simulink model "BGOnly2"  (R2017b)
settings: Solver=VariableStepAuto  StartTime=0.0  StopTime=60  RelTol=1e-3  EnableMultiTasking=on
values from neighbouring files (symbols this model uses):
  beta_str_ch = 0.5*ones(1,5)    [BGOnly2SwitchTest.m]    (also in BGOnlyVar.mat = [0.5 0.5 0.5 0.5 0.5]; PlotBGOnly2.m)
  nu_gpe = 1    [BGOnlyVar.mat]
  nu_gpi = 1    [BGOnlyVar.mat]
  nu_stn = 1    [BGOnlyVar.mat]
  nu_str = 1    [BGOnlyVar.mat]
  teta = 0.02    [BGOnlyVar.mat]
  w_e = 0.9    [BGOnlyVar.mat]
  w_g = 1    [BGOnlyVar.mat]
  w_inh = 0    [BGOnlyVar.mat]
  w_minus = 1    [BGOnlyVar.mat]
  w_plus = 0.9    [BGOnlyVar.mat]
  w_s = 1    [BGOnlyVar.mat]
  w_t = 0.9    [BGOnlyVar.mat]
undefined symbols (not defined in the file or in its folder): sigbuilder_block
libraries: fuzblock x25, simulink x8
settings Model: Creator=User  LastModifiedBy=acaso
settings DataIOCC: LimitDataPoints=on
settings OptimizationCC: LifeSpan=inf
settings DebuggingCC: AllowSymbolicDim=off  SFUnexpectedBacktrackingDiag=warning  SFNoUnconditionalDefaultTransitionDiag=warning  SFExecutionAtInitializationDiag=none
settings ModelReferenceCC: PropagateSignalLabelsOutOfModel=off
settings CodeAppCC: StateflowObjectComments=on
settings GRTTargetCC: TargetLangStandard=C89/C90 (ANSI)
settings ConfigComp: CovMetricSettings=dw  CovHtmlReporting=on  CovSaveCumulativeToWorkspaceVar=on  CovSaveSingleToWorkspaceVar=on  CovExternalEMLEnable=off

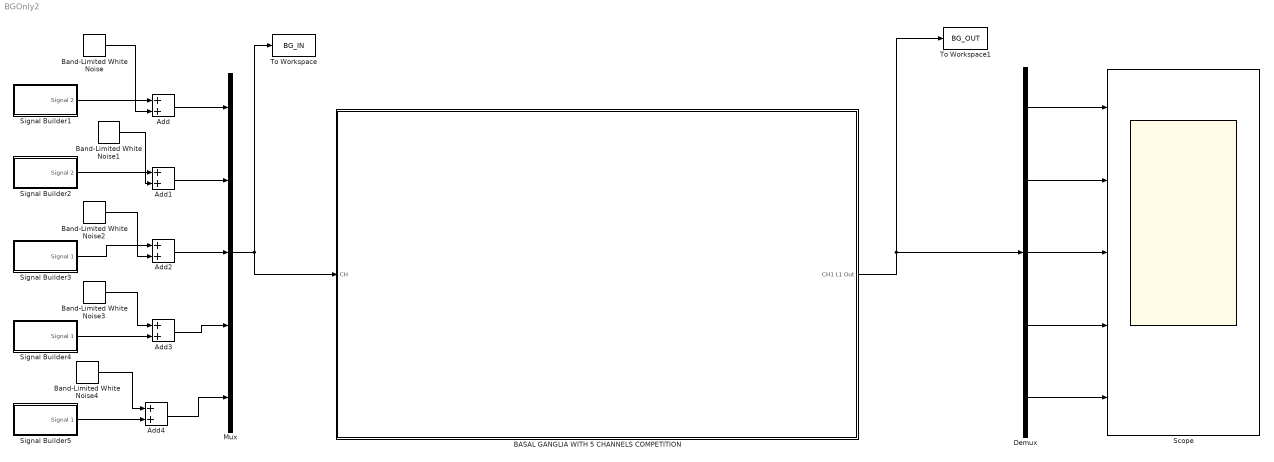
== system BGOnly2 ==
  Add{,1..4} (5 alike) : Sum
  BASAL GANGLIA WITH 5 CHANNELS COMPETITION : Subsystem
  Band-Limited White Noise{,1..4} (5 alike) : simulink/Sources/Band-Limited White Noise  Cov=CHNoise  Ts=0.1  seed=[23341]
  Demux : Demux  Outputs=5
  Mux : Mux  Inputs=5
  Scope : Scope  NumInputPorts=5
  Signal Builder1 : Subsystem  Tag=STV Subsys  LoadFcn=sigbuilder_block('load');  StartFcn=sigbuilder_block('start');  StopFcn=sigbuilder_block('stop');  ClipboardFcn=sigbuilder_block('clipboard');  mask(Sigbuilder block){tuvar=[0:10]}
      mask help: Simulink:masks:SigbuilderBlock_MD
      mask init:
      | if ~strcmp(get_param(bdroot(gcbh),'SimulationStatus'),'stopped') tuvar = sigbuilder_block('maskInit'); end
      settings: CopyFcn=sigbuilder_block('copy');  DeleteFcn=sigbuilder_block('delete');  ModelCloseFcn=sigbuilder_block('modelClose');  PreSaveFcn=sigbuilder_block('preSave');  PauseFcn=sigbuilder_block('pause');  ContinueFcn=sigbuilder_block('continue');  NameChangeFcn=sigbuilder_block('namechange');  OpenFcn=sigbuilder_block('open',[5.4 60.6 1141.2 492 ]);  CloseFcn=sigbuilder_block('close');
      mask Display: plot(0, 0, 100, 100,[2, 2, 32, 32, 2], [68, 8, 8, 68, 68],[32, 2], [38, 38], [32, 19, 2],[53, 60, 44], [32, 17, 17, 2],[16, 16, 31, 31]);txt = getActiveGroup(gcbh);text(2, 100, txt,'verticalAlignment', 'top');
  Signal Builder2 : Subsystem  Tag=STV Subsys  LoadFcn=sigbuilder_block('load');  StartFcn=sigbuilder_block('start');  StopFcn=sigbuilder_block('stop');  ClipboardFcn=sigbuilder_block('clipboard');  mask(Sigbuilder block){tuvar=[0:10]}
      mask help: Simulink:masks:SigbuilderBlock_MD
      mask init:
      | if ~strcmp(get_param(bdroot(gcbh),'SimulationStatus'),'stopped') tuvar = sigbuilder_block('maskInit'); end
      settings: CopyFcn=sigbuilder_block('copy');  DeleteFcn=sigbuilder_block('delete');  ModelCloseFcn=sigbuilder_block('modelClose');  PreSaveFcn=sigbuilder_block('preSave');  PauseFcn=sigbuilder_block('pause');  ContinueFcn=sigbuilder_block('continue');  NameChangeFcn=sigbuilder_block('namechange');  OpenFcn=sigbuilder_block('open',[223.8 139.8 727.2 446.4 ]);  CloseFcn=sigbuilder_block('close');
      mask Display: plot(0, 0, 100, 100,[2, 2, 32, 32, 2], [68, 8, 8, 68, 68],[32, 2], [38, 38], [32, 19, 2],[53, 60, 44], [32, 17, 17, 2],[16, 16, 31, 31]);txt = getActiveGroup(gcbh);text(2, 100, txt,'verticalAlignment', 'top');
  Signal Builder3 : Subsystem  Tag=STV Subsys  LoadFcn=sigbuilder_block('load');  StartFcn=sigbuilder_block('start');  StopFcn=sigbuilder_block('stop');  ClipboardFcn=sigbuilder_block('clipboard');  mask(Sigbuilder block){tuvar=[0:10]}
      mask help: Simulink:masks:SigbuilderBlock_MD
      mask init:
      | if ~strcmp(get_param(bdroot(gcbh),'SimulationStatus'),'stopped') tuvar = sigbuilder_block('maskInit'); end
      settings: CopyFcn=sigbuilder_block('copy');  DeleteFcn=sigbuilder_block('delete');  ModelCloseFcn=sigbuilder_block('modelClose');  PreSaveFcn=sigbuilder_block('preSave');  PauseFcn=sigbuilder_block('pause');  ContinueFcn=sigbuilder_block('continue');  NameChangeFcn=sigbuilder_block('namechange');  OpenFcn=sigbuilder_block('open',[216.6 86.4 727.8 484.8 ]);  CloseFcn=sigbuilder_block('close');
      mask Display: plot(0, 0, 100, 100,[2, 2, 32, 32, 2], [68, 8, 8, 68, 68],[32, 2], [38, 38], [32, 19, 2],[53, 60, 44], [32, 17, 17, 2],[16, 16, 31, 31]);txt = getActiveGroup(gcbh);text(2, 100, txt,'verticalAlignment', 'top');
  Signal Builder4 : Subsystem  Tag=STV Subsys  LoadFcn=sigbuilder_block('load');  StartFcn=sigbuilder_block('start');  StopFcn=sigbuilder_block('stop');  ClipboardFcn=sigbuilder_block('clipboard');  mask(Sigbuilder block){tuvar=[0:10]}
      mask help: Simulink:masks:SigbuilderBlock_MD
      mask init:
      | if ~strcmp(get_param(bdroot(gcbh),'SimulationStatus'),'stopped') tuvar = sigbuilder_block('maskInit'); end
      settings: CopyFcn=sigbuilder_block('copy');  DeleteFcn=sigbuilder_block('delete');  ModelCloseFcn=sigbuilder_block('modelClose');  PreSaveFcn=sigbuilder_block('preSave');  PauseFcn=sigbuilder_block('pause');  ContinueFcn=sigbuilder_block('continue');  NameChangeFcn=sigbuilder_block('namechange');  OpenFcn=sigbuilder_block('open',[216.75 86.25 727.5 485.25 ]);  CloseFcn=sigbuilder_block('close');
      mask Display: plot(0, 0, 100, 100,[2, 2, 32, 32, 2], [68, 8, 8, 68, 68],[32, 2], [38, 38], [32, 19, 2],[53, 60, 44], [32, 17, 17, 2],[16, 16, 31, 31]);txt = getActiveGroup(gcbh);text(2, 100, txt,'verticalAlignment', 'top');
  Signal Builder5 : Subsystem  Tag=STV Subsys  LoadFcn=sigbuilder_block('load');  StartFcn=sigbuilder_block('start');  StopFcn=sigbuilder_block('stop');  ClipboardFcn=sigbuilder_block('clipboard');  mask(Sigbuilder block){tuvar=[0:10]}
      mask help: Simulink:masks:SigbuilderBlock_MD
      mask init:
      | if ~strcmp(get_param(bdroot(gcbh),'SimulationStatus'),'stopped') tuvar = sigbuilder_block('maskInit'); end
      settings: CopyFcn=sigbuilder_block('copy');  DeleteFcn=sigbuilder_block('delete');  ModelCloseFcn=sigbuilder_block('modelClose');  PreSaveFcn=sigbuilder_block('preSave');  PauseFcn=sigbuilder_block('pause');  ContinueFcn=sigbuilder_block('continue');  NameChangeFcn=sigbuilder_block('namechange');  OpenFcn=sigbuilder_block('open',[216.75 86.25 727.5 485.25 ]);  CloseFcn=sigbuilder_block('close');
      mask Display: plot(0, 0, 100, 100,[2, 2, 32, 32, 2], [68, 8, 8, 68, 68],[32, 2], [38, 38], [32, 19, 2],[53, 60, 44], [32, 17, 17, 2],[16, 16, 31, 31]);txt = getActiveGroup(gcbh);text(2, 100, txt,'verticalAlignment', 'top');
  To Workspace : ToWorkspace  VariableName=BG_IN  SaveFormat=Timeseries  SampleTime=0.1
  To Workspace1 : ToWorkspace  VariableName=BG_OUT  SaveFormat=Timeseries  SampleTime=0.1
  wires:
  Mux/1 -> To Workspace/1, BASAL GANGLIA WITH 5 CHANNELS COMPETITION/1("CH ")
  BASAL GANGLIA WITH 5 CHANNELS COMPETITION/1(CH1 L1 Out) -> To Workspace1/1, Demux/1
  Demux/5 -> Scope/5
  Demux/4 -> Scope/4
  Demux/3 -> Scope/3
  Demux/2 -> Scope/2
  Demux/1 -> Scope/1
  Signal Builder1/1(Signal 2) -> Add/1
  Add/1 -> Mux/1
  Band-Limited White Noise/1 -> Add/2
  Add1/1 -> Mux/2
  Signal Builder2/1(Signal 2) -> Add1/1
  Band-Limited White Noise1/1 -> Add1/2
  Add2/1 -> Mux/3
  Signal Builder3/1(Signal 1) -> Add2/1
  Band-Limited White Noise2/1 -> Add2/2
  Add3/1 -> Mux/4
  Signal Builder4/1(Signal 1) -> Add3/2
  Band-Limited White Noise3/1 -> Add3/1
  Add4/1 -> Mux/5
  Signal Builder5/1(Signal 1) -> Add4/2
  Band-Limited White Noise4/1 -> Add4/1

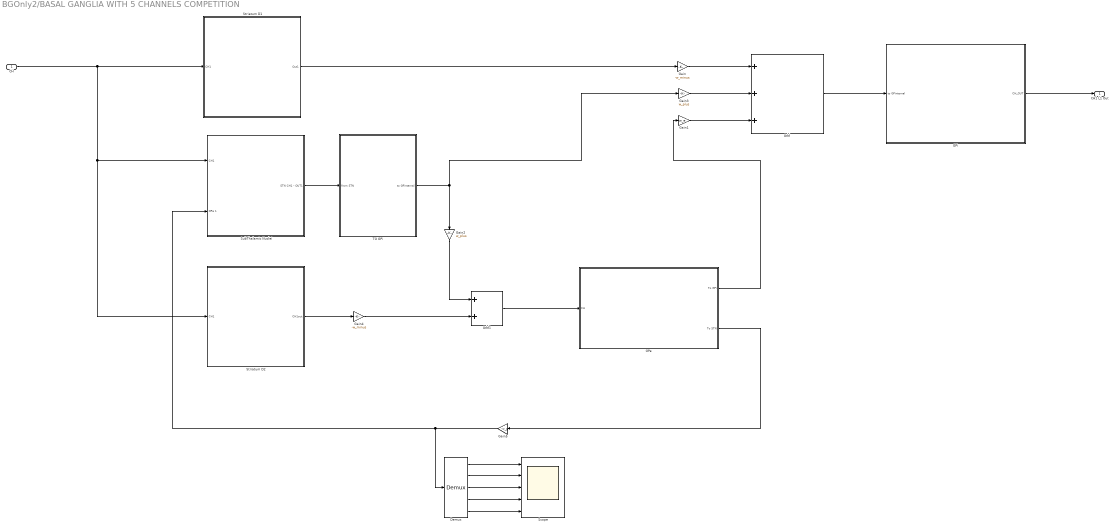
== system BGOnly2/BASAL GANGLIA WITH 5 CHANNELS COMPETITION ==
  "CH " : Inport
  Add : Sum  Inputs=3
  Add1 : Sum  Inputs=2
  Demux : Demux  Outputs=5
  GPe : Subsystem  TreatAsAtomicUnit=on
  GPi : Subsystem
  Gain : Gain  Gain=-w_minus
  Gain1 : Gain  Gain=w_e
  Gain2 : Gain  Gain=w_plus
  Gain3 : Gain  Gain=w_plus
  Gain4 : Gain  Gain=-w_minus
  Gain5 : Gain  Gain=-w_g
  Scope : Scope  NumInputPorts=5
  "Striatum D1 " : Subsystem
  Striatum D2 : Subsystem
  SubThalamic Nuclei : Subsystem
  TO GPi : Subsystem
  CH1 L1 Out : Outport
  wires:
  TO GPi/1(to GPinternal) -> Gain3/1, Gain2/1
  GPi/1("CH_OUT ") -> CH1 L1 Out/1
  "CH "/1 -> Striatum D2/1(CH1), SubThalamic Nuclei/1(CH1), "Striatum D1 "/1(CH1)
  "Striatum D1 "/1(Out1) -> Gain/1
  SubThalamic Nuclei/1(STN CH1 - OUT1) -> TO GPi/1("from STN ")
  GPe/1(To GPi) -> Gain1/1
  Gain/1 -> Add/1
  Gain3/1 -> Add/2
  Gain1/1 -> Add/3
  Striatum D2/1(CH1out) -> Gain4/1
  Gain2/1 -> Add1/1
  Gain4/1 -> Add1/2
  Add1/1 -> GPe/1(CH)
  GPe/2(To STN) -> Gain5/1
  Gain5/1 -> Demux/1, SubThalamic Nuclei/2(GPe 1)
  Add/1 -> GPi/1("to GPinternal ")
  Demux/1 -> Scope/1
  Demux/2 -> Scope/2
  Demux/3 -> Scope/3
  Demux/4 -> Scope/4
  Demux/5 -> Scope/5

== system BGOnly2/Signal Builder1 ==
  Demux : Demux  Tag=STV Demux  Outputs=1
  FromWs : FromWorkspace  Tag=STV FromWs  VariableName=tuvar  SampleTime=0
      SigBuilderData=|
      | common.afterFinalStr = 'Extrapolate'
      | common.sampleTime = 0
      | dataSet.timeRange = [0 60]
      | dataSet.name = 'Group 1'
      | sbobj.Groups.Name = 'Group 1'
      | sbobj.Groups.Signals.Name = 'Signal 2'
      | sbobj.Groups.Signals.XData = [0 20.1 20.1 29.5 30.4 40.1 40.1 59.7 60]
      | sbobj.Groups.Signals.YData = [0 0 1 1 0.8 0.795 0.005 0.0001 0.0001]
      | sbobj.Groups.TimeRange = [0 60]
  Signal 2 : Outport  Tag=STV Outport
  wires:
  FromWs/1 -> Demux/1
  Demux/1 -> Signal 2/1

== system BGOnly2/Signal Builder2 ==
  Demux : Demux  Tag=STV Demux  Outputs=1
  FromWs : FromWorkspace  Tag=STV FromWs  VariableName=tuvar  SampleTime=0
      SigBuilderData=|
      | common.afterFinalStr = 'Extrapolate'
      | common.sampleTime = 0
      | dataSet.timeRange = [0 60]
      | dataSet.name = 'Group 1'
      | sbobj.Groups.Name = 'Group 1'
      | sbobj.Groups.Signals.Name = 'Signal 2'
      | sbobj.Groups.Signals.XData = [0 30.1 30.1 39.7 40.4 49.9 49.9 60]
      | sbobj.Groups.Signals.YData = [0 0 0.8 0.795 1 1 0 0]
      | sbobj.Groups.TimeRange = [0 60]
  Signal 2 : Outport  Tag=STV Outport
  wires:
  FromWs/1 -> Demux/1
  Demux/1 -> Signal 2/1

== system BGOnly2/Signal Builder3 ==
  Demux : Demux  Tag=STV Demux  Outputs=1
  FromWs : FromWorkspace  Tag=STV FromWs  VariableName=tuvar  SampleTime=0
      SigBuilderData=|
      | common.afterFinalStr = 'Extrapolate'
      | common.sampleTime = 0
      | dataSet.timeRange = [0 60]
      | dataSet.name = 'Group 1'
      | sbobj.Groups.Name = 'Group 1'
      | sbobj.Groups.Signals.Name = 'Signal 1'
      | sbobj.Groups.Signals.XData = [0 60]
      | sbobj.Groups.Signals.YData = [0 0]
      | sbobj.Groups.TimeRange = [0 60]
  Signal 1 : Outport  Tag=STV Outport
  wires:
  FromWs/1 -> Demux/1
  Demux/1 -> Signal 1/1

== system BGOnly2/Signal Builder4 ==
  Demux : Demux  Tag=STV Demux  Outputs=1
  FromWs : FromWorkspace  Tag=STV FromWs  VariableName=tuvar  SampleTime=0
      SigBuilderData=|
      | common.afterFinalStr = 'Extrapolate'
      | common.sampleTime = 0
      | dataSet.timeRange = [0 60]
      | dataSet.name = 'Group 1'
      | sbobj.Groups.Name = 'Group 1'
      | sbobj.Groups.Signals.Name = 'Signal 1'
      | sbobj.Groups.Signals.XData = [0 60]
      | sbobj.Groups.Signals.YData = [0 0]
      | sbobj.Groups.TimeRange = [0 60]
  Signal 1 : Outport  Tag=STV Outport
  wires:
  FromWs/1 -> Demux/1
  Demux/1 -> Signal 1/1

== system BGOnly2/Signal Builder5 ==
  Demux : Demux  Tag=STV Demux  Outputs=1
  FromWs : FromWorkspace  Tag=STV FromWs  VariableName=tuvar  SampleTime=0
      SigBuilderData=|
      | common.afterFinalStr = 'Extrapolate'
      | common.sampleTime = 0
      | dataSet.timeRange = [0 60]
      | dataSet.name = 'Group 1'
      | sbobj.Groups.Name = 'Group 1'
      | sbobj.Groups.Signals.Name = 'Signal 1'
      | sbobj.Groups.Signals.XData = [0 60]
      | sbobj.Groups.Signals.YData = [0 0]
      | sbobj.Groups.TimeRange = [0 60]
  Signal 1 : Outport  Tag=STV Outport
  wires:
  FromWs/1 -> Demux/1
  Demux/1 -> Signal 1/1

== system BGOnly2/BASAL GANGLIA WITH 5 CHANNELS COMPETITION/GPe ==
  CH : Inport
  GPe CH1 : Subsystem
  To GPi : Outport
  To STN : Outport  Port=2
  wires:
  CH/1 -> GPe CH1/1(In)
  GPe CH1/1(To GPi) -> To GPi/1
  GPe CH1/2(To STN) -> To STN/1

== system BGOnly2/BASAL GANGLIA WITH 5 CHANNELS COMPETITION/GPi ==
  "to GPinternal " : Inport
  GPinternal : Subsystem
  "CH_OUT " : Outport
  wires:
  "to GPinternal "/1 -> GPinternal/1("to GPinternal ")
  GPinternal/1(To Thal) -> "CH_OUT "/1

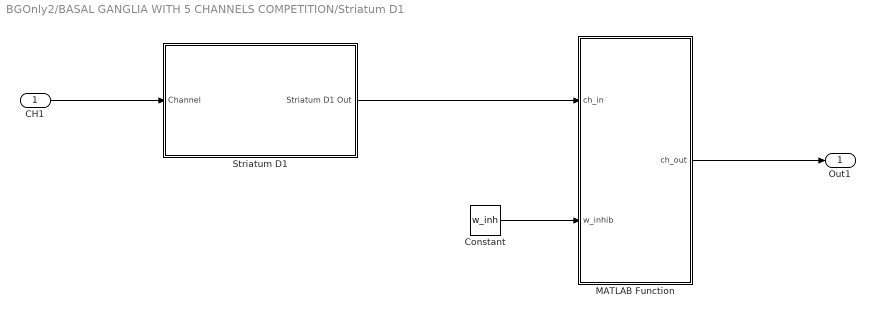
== system BGOnly2/BASAL GANGLIA WITH 5 CHANNELS COMPETITION/Striatum D1  ==
  CH1 : Inport
  Constant : Constant  Value=w_inh
  MATLAB Function : MATLAB Function  TreatAsAtomicUnit=on
  "Striatum D1 " : Subsystem
  Out1 : Outport
  wires:
  CH1/1 -> "Striatum D1 "/1(Channel)
  "Striatum D1 "/1(Striatum D1 Out) -> MATLAB Function/1(ch_in)
  Constant/1 -> MATLAB Function/2(w_inhib)
  MATLAB Function/1(ch_out) -> Out1/1

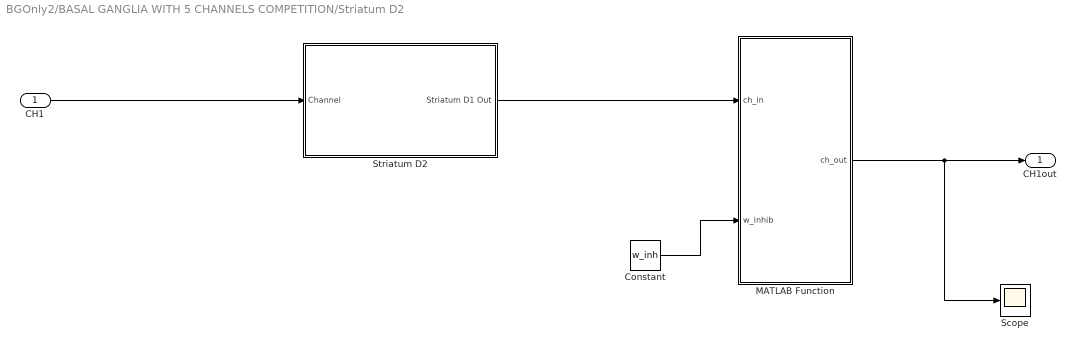
== system BGOnly2/BASAL GANGLIA WITH 5 CHANNELS COMPETITION/Striatum D2 ==
  CH1 : Inport
  Constant : Constant  Value=w_inh
  MATLAB Function : MATLAB Function  TreatAsAtomicUnit=on
  Scope : Scope
  "Striatum D2 " : Subsystem
  CH1out : Outport
  wires:
  MATLAB Function/1(ch_out) -> Scope/1, CH1out/1
  CH1/1 -> "Striatum D2 "/1(Channel)
  "Striatum D2 "/1(Striatum D1 Out) -> MATLAB Function/1(ch_in)
  Constant/1 -> MATLAB Function/2(w_inhib)

== system BGOnly2/BASAL GANGLIA WITH 5 CHANNELS COMPETITION/SubThalamic Nuclei ==
  CH1 : Inport
  GPe 1 : Inport  Port=2
  "SubThalamic Nucleus (STN) " : Subsystem
  STN CH1 - OUT1 : Outport
  wires:
  CH1/1 -> "SubThalamic Nucleus (STN) "/1(Channel)
  GPe 1/1 -> "SubThalamic Nucleus (STN) "/2(GPe Inp)
  "SubThalamic Nucleus (STN) "/1(STN Out1) -> STN CH1 - OUT1/1

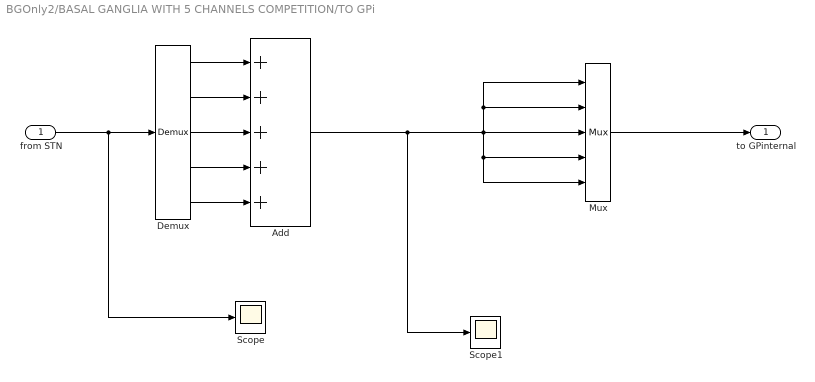
== system BGOnly2/BASAL GANGLIA WITH 5 CHANNELS COMPETITION/TO GPi ==
  "from STN " : Inport
  Add : Sum  Inputs=5
  Demux : Demux  Outputs=5
  Mux : Mux  Inputs=5
  Scope : Scope
  Scope1 : Scope
  to GPinternal : Outport
  wires:
  "from STN "/1 -> Scope/1, Demux/1
  Demux/1 -> Add/1
  Demux/2 -> Add/2
  Demux/3 -> Add/3
  Demux/4 -> Add/4
  Demux/5 -> Add/5
  Add/1 -> Scope1/1, Mux/1, Mux/2, Mux/3, Mux/4, Mux/5
  Mux/1 -> to GPinternal/1

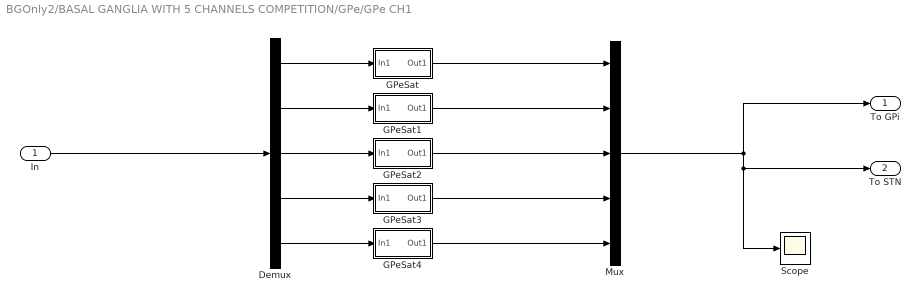
== system BGOnly2/BASAL GANGLIA WITH 5 CHANNELS COMPETITION/GPe/GPe CH1 ==
  In : Inport
  Demux : Demux  Outputs=5
  GPeSat : Subsystem
  GPeSat1 : Subsystem
  GPeSat2 : Subsystem
  GPeSat3 : Subsystem
  GPeSat4 : Subsystem
  Mux : Mux  Inputs=5
  Scope : Scope
  To GPi : Outport
  To STN : Outport  Port=2
  wires:
  Mux/1 -> To STN/1, Scope/1, To GPi/1
  Demux/1 -> GPeSat/1(In1)
  GPeSat/1(Out1) -> Mux/1
  Demux/2 -> GPeSat1/1(In1)
  GPeSat1/1(Out1) -> Mux/2
  Demux/3 -> GPeSat2/1(In1)
  GPeSat2/1(Out1) -> Mux/3
  Demux/4 -> GPeSat3/1(In1)
  GPeSat3/1(Out1) -> Mux/4
  Demux/5 -> GPeSat4/1(In1)
  GPeSat4/1(Out1) -> Mux/5
  In/1 -> Demux/1

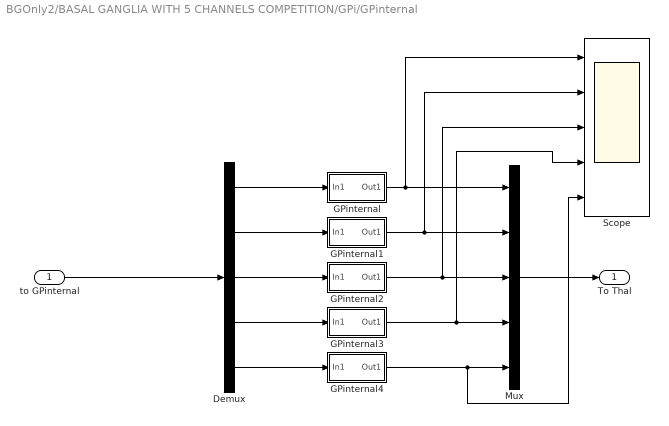
== system BGOnly2/BASAL GANGLIA WITH 5 CHANNELS COMPETITION/GPi/GPinternal ==
  "to GPinternal " : Inport
  Demux : Demux  Outputs=5
  GPinternal : Subsystem
  GPinternal1 : Subsystem
  GPinternal2 : Subsystem
  GPinternal3 : Subsystem
  GPinternal4 : Subsystem
  Mux : Mux  Inputs=5
  Scope : Scope  NumInputPorts=5
  To Thal : Outport
  wires:
  Demux/1 -> GPinternal/1(In1)
  GPinternal/1(Out1) -> Mux/1, Scope/1
  Demux/2 -> GPinternal1/1(In1)
  Demux/3 -> GPinternal2/1(In1)
  GPinternal2/1(Out1) -> Scope/3, Mux/3
  Demux/4 -> GPinternal3/1(In1)
  GPinternal3/1(Out1) -> Scope/4, Mux/4
  Demux/5 -> GPinternal4/1(In1)
  GPinternal4/1(Out1) -> Scope/5, Mux/5
  "to GPinternal "/1 -> Demux/1
  Mux/1 -> To Thal/1
  GPinternal1/1(Out1) -> Scope/2, Mux/2

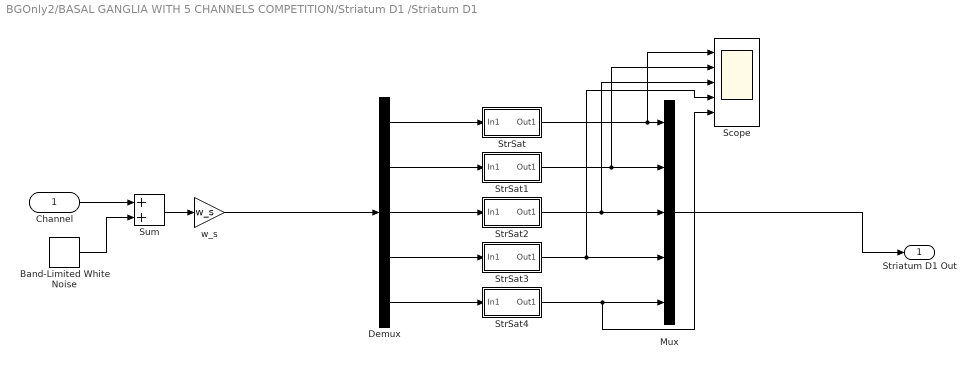
== system BGOnly2/BASAL GANGLIA WITH 5 CHANNELS COMPETITION/Striatum D1 /Striatum D1  ==
  Channel : Inport
  Band-Limited White Noise : simulink/Sources/Band-Limited White Noise  Cov=[0]  Ts=0.1  seed=[23341]
  Demux : Demux  Outputs=5
  Mux : Mux  Inputs=5
  Scope : Scope  NumInputPorts=5
  StrSat : Subsystem
  StrSat1 : Subsystem
  StrSat2 : Subsystem
  StrSat3 : Subsystem
  StrSat4 : Subsystem
  Sum : Sum
  w_s : Gain  Gain=w_s
  Striatum D1 Out : Outport
  wires:
  Channel/1 -> Sum/1
  Sum/1 -> w_s/1
  Mux/1 -> Striatum D1 Out/1
  Band-Limited White Noise/1 -> Sum/2
  Demux/1 -> StrSat/1(In1)
  StrSat/1(Out1) -> Scope/1, Mux/1
  Demux/2 -> StrSat1/1(In1)
  StrSat1/1(Out1) -> Scope/2, Mux/2
  Demux/3 -> StrSat2/1(In1)
  StrSat2/1(Out1) -> Scope/3, Mux/3
  Demux/4 -> StrSat3/1(In1)
  StrSat3/1(Out1) -> Scope/4, Mux/4
  Demux/5 -> StrSat4/1(In1)
  w_s/1 -> Demux/1
  StrSat4/1(Out1) -> Scope/5, Mux/5

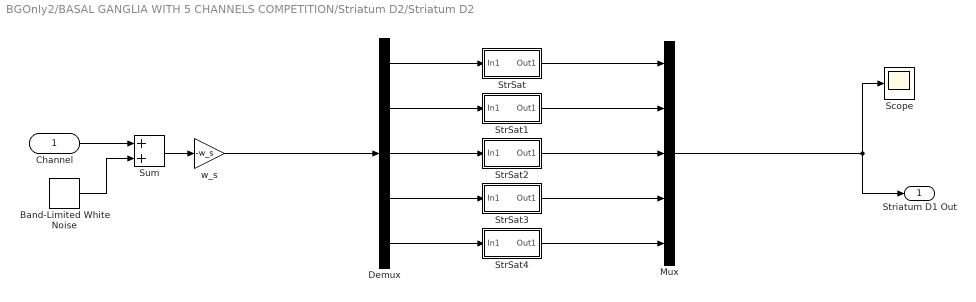
== system BGOnly2/BASAL GANGLIA WITH 5 CHANNELS COMPETITION/Striatum D2/Striatum D2  ==
  Channel : Inport
  Band-Limited White Noise : simulink/Sources/Band-Limited White Noise  Cov=[0]  Ts=0.1  seed=[23341]
  Demux : Demux  Outputs=5
  Mux : Mux  Inputs=5
  Scope : Scope
  StrSat : Subsystem
  StrSat1 : Subsystem
  StrSat2 : Subsystem
  StrSat3 : Subsystem
  StrSat4 : Subsystem
  Sum : Sum
  w_s : Gain  Gain=-w_s
  Striatum D1 Out : Outport
  wires:
  Channel/1 -> Sum/1
  Sum/1 -> w_s/1
  Mux/1 -> Striatum D1 Out/1, Scope/1
  Band-Limited White Noise/1 -> Sum/2
  Demux/1 -> StrSat/1(In1)
  StrSat/1(Out1) -> Mux/1
  Demux/2 -> StrSat1/1(In1)
  StrSat1/1(Out1) -> Mux/2
  Demux/3 -> StrSat2/1(In1)
  StrSat2/1(Out1) -> Mux/3
  Demux/4 -> StrSat3/1(In1)
  StrSat3/1(Out1) -> Mux/4
  Demux/5 -> StrSat4/1(In1)
  StrSat4/1(Out1) -> Mux/5
  w_s/1 -> Demux/1

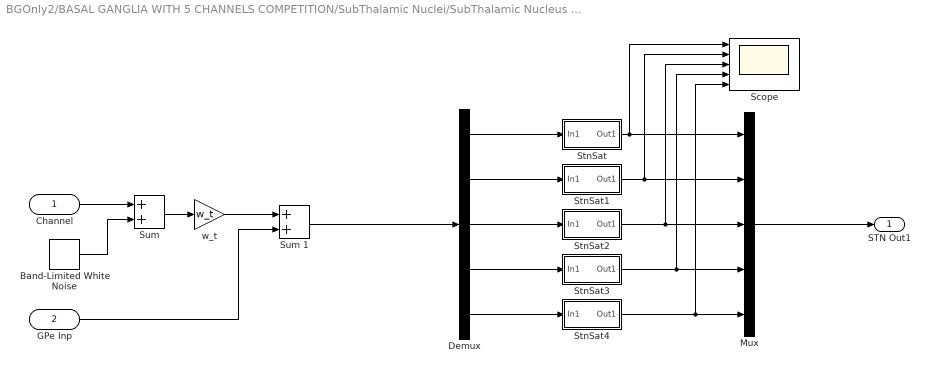
== system BGOnly2/BASAL GANGLIA WITH 5 CHANNELS COMPETITION/SubThalamic Nuclei/SubThalamic Nucleus (STN)  ==
  Channel : Inport
  GPe Inp : Inport  Port=2
  Band-Limited White Noise : simulink/Sources/Band-Limited White Noise  Cov=[0]  Ts=0.1  seed=[23341]
  Demux : Demux  Outputs=5
  Mux : Mux  Inputs=5
  Scope : Scope  NumInputPorts=5
  StnSat : Subsystem
  StnSat1 : Subsystem
  StnSat2 : Subsystem
  StnSat3 : Subsystem
  StnSat4 : Subsystem
  "Sum " : Sum
  Sum 1 : Sum
  w_t : Gain  Gain=w_t
  STN Out1 : Outport
  wires:
  w_t/1 -> Sum 1/1
  Channel/1 -> "Sum "/1
  Band-Limited White Noise/1 -> "Sum "/2
  "Sum "/1 -> w_t/1
  GPe Inp/1 -> Sum 1/2
  Mux/1 -> STN Out1/1
  Demux/1 -> StnSat/1(In1)
  Demux/2 -> StnSat1/1(In1)
  StnSat1/1(Out1) -> Scope/2, Mux/2
  Demux/3 -> StnSat2/1(In1)
  StnSat2/1(Out1) -> Scope/3, Mux/3
  Demux/4 -> StnSat3/1(In1)
  StnSat3/1(Out1) -> Scope/4, Mux/4
  Demux/5 -> StnSat4/1(In1)
  StnSat4/1(Out1) -> Scope/5, Mux/5
  Sum 1/1 -> Demux/1
  StnSat/1(Out1) -> Scope/1, Mux/1

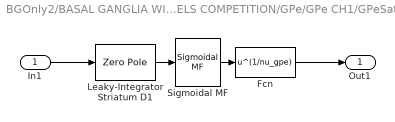
== system BGOnly2/BASAL GANGLIA WITH 5 CHANNELS COMPETITION/GPe/GPe CH1/GPeSat ==
  In1 : Inport
  Fcn : Fcn  Expr=u^(1/nu_gpe)
  "Leaky-Integrator Striatum D1 " : ZeroPole  Zeros=[]  Poles=[-1/teta]  Gain=[1.5/teta]
  Sigmoidal MF : fuzblock/Membership  Functions/Sigmoidal MF  a=alpha_gpe  c=beta_gpe
      settings: SourceProductName=Fuzzy Logic Toolbox  SourceProductBaseCode=FL
  Out1 : Outport
  wires:
  Fcn/1 -> Out1/1
  Sigmoidal MF/1 -> Fcn/1
  "Leaky-Integrator Striatum D1 "/1 -> Sigmoidal MF/1
  In1/1 -> "Leaky-Integrator Striatum D1 "/1

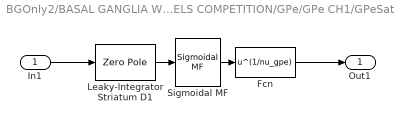
== system BGOnly2/BASAL GANGLIA WITH 5 CHANNELS COMPETITION/GPe/GPe CH1/GPeSat1 ==
  In1 : Inport
  Fcn : Fcn  Expr=u^(1/nu_gpe)
  "Leaky-Integrator Striatum D1 " : ZeroPole  Zeros=[]  Poles=[-1/teta]  Gain=[1.5/teta]
  Sigmoidal MF : fuzblock/Membership  Functions/Sigmoidal MF  a=alpha_gpe  c=beta_gpe
      settings: SourceProductName=Fuzzy Logic Toolbox  SourceProductBaseCode=FL
  Out1 : Outport
  wires:
  Fcn/1 -> Out1/1
  Sigmoidal MF/1 -> Fcn/1
  "Leaky-Integrator Striatum D1 "/1 -> Sigmoidal MF/1
  In1/1 -> "Leaky-Integrator Striatum D1 "/1

== system BGOnly2/BASAL GANGLIA WITH 5 CHANNELS COMPETITION/GPe/GPe CH1/GPeSat2 ==
  In1 : Inport
  Fcn : Fcn  Expr=u^(1/nu_gpe)
  "Leaky-Integrator Striatum D1 " : ZeroPole  Zeros=[]  Poles=[-1/teta]  Gain=[1.5/teta]
  Sigmoidal MF : fuzblock/Membership  Functions/Sigmoidal MF  a=alpha_gpe  c=beta_gpe
      settings: SourceProductName=Fuzzy Logic Toolbox  SourceProductBaseCode=FL
  Out1 : Outport
  wires:
  Fcn/1 -> Out1/1
  Sigmoidal MF/1 -> Fcn/1
  "Leaky-Integrator Striatum D1 "/1 -> Sigmoidal MF/1
  In1/1 -> "Leaky-Integrator Striatum D1 "/1

== system BGOnly2/BASAL GANGLIA WITH 5 CHANNELS COMPETITION/GPe/GPe CH1/GPeSat3 ==
  In1 : Inport
  Fcn : Fcn  Expr=u^(1/nu_gpe)
  "Leaky-Integrator Striatum D1 " : ZeroPole  Zeros=[]  Poles=[-1/teta]  Gain=[1.5/teta]
  Sigmoidal MF : fuzblock/Membership  Functions/Sigmoidal MF  a=alpha_gpe  c=beta_gpe
      settings: SourceProductName=Fuzzy Logic Toolbox  SourceProductBaseCode=FL
  Out1 : Outport
  wires:
  Fcn/1 -> Out1/1
  Sigmoidal MF/1 -> Fcn/1
  "Leaky-Integrator Striatum D1 "/1 -> Sigmoidal MF/1
  In1/1 -> "Leaky-Integrator Striatum D1 "/1

== system BGOnly2/BASAL GANGLIA WITH 5 CHANNELS COMPETITION/GPe/GPe CH1/GPeSat4 ==
  In1 : Inport
  Fcn : Fcn  Expr=u^(1/nu_gpe)
  "Leaky-Integrator Striatum D1 " : ZeroPole  Zeros=[]  Poles=[-1/teta]  Gain=[1.5/teta]
  Sigmoidal MF : fuzblock/Membership  Functions/Sigmoidal MF  a=alpha_gpe  c=beta_gpe
      settings: SourceProductName=Fuzzy Logic Toolbox  SourceProductBaseCode=FL
  Out1 : Outport
  wires:
  Fcn/1 -> Out1/1
  Sigmoidal MF/1 -> Fcn/1
  "Leaky-Integrator Striatum D1 "/1 -> Sigmoidal MF/1
  In1/1 -> "Leaky-Integrator Striatum D1 "/1

== system BGOnly2/BASAL GANGLIA WITH 5 CHANNELS COMPETITION/GPi/GPinternal/GPinternal ==
  In1 : Inport
  Fcn : Fcn  Expr=u^(1/nu_gpi)
  "Leaky-Integrator Striatum D1 " : ZeroPole  Zeros=[]  Poles=[-1/teta]  Gain=[1.5/teta]
  Sigmoidal MF : fuzblock/Membership  Functions/Sigmoidal MF  a=alpha_gpi  c=beta_gpi
      settings: SourceProductName=Fuzzy Logic Toolbox  SourceProductBaseCode=FL
  Out1 : Outport
  wires:
  Fcn/1 -> Out1/1
  Sigmoidal MF/1 -> Fcn/1
  "Leaky-Integrator Striatum D1 "/1 -> Sigmoidal MF/1
  In1/1 -> "Leaky-Integrator Striatum D1 "/1

== system BGOnly2/BASAL GANGLIA WITH 5 CHANNELS COMPETITION/GPi/GPinternal/GPinternal1 ==
  In1 : Inport
  Fcn : Fcn  Expr=u^(1/nu_gpi)
  "Leaky-Integrator Striatum D1 " : ZeroPole  Zeros=[]  Poles=[-1/teta]  Gain=[1.5/teta]
  Sigmoidal MF : fuzblock/Membership  Functions/Sigmoidal MF  a=alpha_gpi  c=beta_gpi
      settings: SourceProductName=Fuzzy Logic Toolbox  SourceProductBaseCode=FL
  Out1 : Outport
  wires:
  Fcn/1 -> Out1/1
  Sigmoidal MF/1 -> Fcn/1
  "Leaky-Integrator Striatum D1 "/1 -> Sigmoidal MF/1
  In1/1 -> "Leaky-Integrator Striatum D1 "/1

== system BGOnly2/BASAL GANGLIA WITH 5 CHANNELS COMPETITION/GPi/GPinternal/GPinternal2 ==
  In1 : Inport
  Fcn : Fcn  Expr=u^(1/nu_gpi)
  "Leaky-Integrator Striatum D1 " : ZeroPole  Zeros=[]  Poles=[-1/teta]  Gain=[1.5/teta]
  Sigmoidal MF : fuzblock/Membership  Functions/Sigmoidal MF  a=alpha_gpi  c=beta_gpi
      settings: SourceProductName=Fuzzy Logic Toolbox  SourceProductBaseCode=FL
  Out1 : Outport
  wires:
  Fcn/1 -> Out1/1
  Sigmoidal MF/1 -> Fcn/1
  "Leaky-Integrator Striatum D1 "/1 -> Sigmoidal MF/1
  In1/1 -> "Leaky-Integrator Striatum D1 "/1

== system BGOnly2/BASAL GANGLIA WITH 5 CHANNELS COMPETITION/GPi/GPinternal/GPinternal3 ==
  In1 : Inport
  Fcn : Fcn  Expr=u^(1/nu_gpi)
  "Leaky-Integrator Striatum D1 " : ZeroPole  Zeros=[]  Poles=[-1/teta]  Gain=[1.5/teta]
  Sigmoidal MF : fuzblock/Membership  Functions/Sigmoidal MF  a=alpha_gpi  c=beta_gpi
      settings: SourceProductName=Fuzzy Logic Toolbox  SourceProductBaseCode=FL
  Out1 : Outport
  wires:
  Fcn/1 -> Out1/1
  Sigmoidal MF/1 -> Fcn/1
  "Leaky-Integrator Striatum D1 "/1 -> Sigmoidal MF/1
  In1/1 -> "Leaky-Integrator Striatum D1 "/1

== system BGOnly2/BASAL GANGLIA WITH 5 CHANNELS COMPETITION/GPi/GPinternal/GPinternal4 ==
  In1 : Inport
  Fcn : Fcn  Expr=u^(1/nu_gpi)
  "Leaky-Integrator Striatum D1 " : ZeroPole  Zeros=[]  Poles=[-1/teta]  Gain=[1.5/teta]
  Sigmoidal MF : fuzblock/Membership  Functions/Sigmoidal MF  a=alpha_gpi  c=beta_gpi
      settings: SourceProductName=Fuzzy Logic Toolbox  SourceProductBaseCode=FL
  Out1 : Outport
  wires:
  Fcn/1 -> Out1/1
  Sigmoidal MF/1 -> Fcn/1
  "Leaky-Integrator Striatum D1 "/1 -> Sigmoidal MF/1
  In1/1 -> "Leaky-Integrator Striatum D1 "/1

== system BGOnly2/BASAL GANGLIA WITH 5 CHANNELS COMPETITION/Striatum D1 /Striatum D1 /StrSat ==
  In1 : Inport
  Fcn : Fcn  Expr=u^(1/nu_str)
  "Leaky-Integrator Striatum D1 " : ZeroPole  Zeros=[]  Poles=[-1/teta]  Gain=[1.5/teta]
  Sigmoidal MF : fuzblock/Membership  Functions/Sigmoidal MF  a=alpha_str  c=beta_str_ch(1)
      settings: SourceProductName=Fuzzy Logic Toolbox  SourceProductBaseCode=FL
  Out1 : Outport
  wires:
  Fcn/1 -> Out1/1
  Sigmoidal MF/1 -> Fcn/1
  "Leaky-Integrator Striatum D1 "/1 -> Sigmoidal MF/1
  In1/1 -> "Leaky-Integrator Striatum D1 "/1

== system BGOnly2/BASAL GANGLIA WITH 5 CHANNELS COMPETITION/Striatum D1 /Striatum D1 /StrSat1 ==
  In1 : Inport
  Fcn : Fcn  Expr=u^(1/nu_str)
  "Leaky-Integrator Striatum D1 " : ZeroPole  Zeros=[]  Poles=[-1/teta]  Gain=[1.5/teta]
  Sigmoidal MF : fuzblock/Membership  Functions/Sigmoidal MF  a=alpha_str  c=beta_str_ch(2)
      settings: SourceProductName=Fuzzy Logic Toolbox  SourceProductBaseCode=FL
  Out1 : Outport
  wires:
  Fcn/1 -> Out1/1
  Sigmoidal MF/1 -> Fcn/1
  "Leaky-Integrator Striatum D1 "/1 -> Sigmoidal MF/1
  In1/1 -> "Leaky-Integrator Striatum D1 "/1

== system BGOnly2/BASAL GANGLIA WITH 5 CHANNELS COMPETITION/Striatum D1 /Striatum D1 /StrSat2 ==
  In1 : Inport
  Fcn : Fcn  Expr=u^(1/nu_str)
  "Leaky-Integrator Striatum D1 " : ZeroPole  Zeros=[]  Poles=[-1/teta]  Gain=[1.5/teta]
  Sigmoidal MF : fuzblock/Membership  Functions/Sigmoidal MF  a=alpha_str  c=beta_str_ch(3)
      settings: SourceProductName=Fuzzy Logic Toolbox  SourceProductBaseCode=FL
  Out1 : Outport
  wires:
  Fcn/1 -> Out1/1
  Sigmoidal MF/1 -> Fcn/1
  "Leaky-Integrator Striatum D1 "/1 -> Sigmoidal MF/1
  In1/1 -> "Leaky-Integrator Striatum D1 "/1

== system BGOnly2/BASAL GANGLIA WITH 5 CHANNELS COMPETITION/Striatum D1 /Striatum D1 /StrSat3 ==
  In1 : Inport
  Fcn : Fcn  Expr=u^(1/nu_str)
  "Leaky-Integrator Striatum D1 " : ZeroPole  Zeros=[]  Poles=[-1/teta]  Gain=[1.5/teta]
  Sigmoidal MF : fuzblock/Membership  Functions/Sigmoidal MF  a=alpha_str  c=beta_str_ch(4)
      settings: SourceProductName=Fuzzy Logic Toolbox  SourceProductBaseCode=FL
  Out1 : Outport
  wires:
  Fcn/1 -> Out1/1
  Sigmoidal MF/1 -> Fcn/1
  "Leaky-Integrator Striatum D1 "/1 -> Sigmoidal MF/1
  In1/1 -> "Leaky-Integrator Striatum D1 "/1

== system BGOnly2/BASAL GANGLIA WITH 5 CHANNELS COMPETITION/Striatum D1 /Striatum D1 /StrSat4 ==
  In1 : Inport
  Fcn : Fcn  Expr=u^(1/nu_str)
  "Leaky-Integrator Striatum D1 " : ZeroPole  Zeros=[]  Poles=[-1/teta]  Gain=[1.5/teta]
  Sigmoidal MF : fuzblock/Membership  Functions/Sigmoidal MF  a=alpha_str  c=beta_str_ch(5)
      settings: SourceProductName=Fuzzy Logic Toolbox  SourceProductBaseCode=FL
  Out1 : Outport
  wires:
  Fcn/1 -> Out1/1
  Sigmoidal MF/1 -> Fcn/1
  "Leaky-Integrator Striatum D1 "/1 -> Sigmoidal MF/1
  In1/1 -> "Leaky-Integrator Striatum D1 "/1

== system BGOnly2/BASAL GANGLIA WITH 5 CHANNELS COMPETITION/Striatum D2/Striatum D2 /StrSat ==
  In1 : Inport
  Fcn : Fcn  Expr=u^(1/nu_str)
  "Leaky-Integrator Striatum D1 " : ZeroPole  Zeros=[]  Poles=[-1/teta]  Gain=[1.5/teta]
  Sigmoidal MF : fuzblock/Membership  Functions/Sigmoidal MF  a=alpha_str  c=beta_str_ch(1)
      settings: SourceProductName=Fuzzy Logic Toolbox  SourceProductBaseCode=FL
  Out1 : Outport
  wires:
  Fcn/1 -> Out1/1
  Sigmoidal MF/1 -> Fcn/1
  "Leaky-Integrator Striatum D1 "/1 -> Sigmoidal MF/1
  In1/1 -> "Leaky-Integrator Striatum D1 "/1

== system BGOnly2/BASAL GANGLIA WITH 5 CHANNELS COMPETITION/Striatum D2/Striatum D2 /StrSat1 ==
  In1 : Inport
  Fcn : Fcn  Expr=u^(1/nu_str)
  "Leaky-Integrator Striatum D1 " : ZeroPole  Zeros=[]  Poles=[-1/teta]  Gain=[1.5/teta]
  Sigmoidal MF : fuzblock/Membership  Functions/Sigmoidal MF  a=alpha_str  c=beta_str_ch(2)
      settings: SourceProductName=Fuzzy Logic Toolbox  SourceProductBaseCode=FL
  Out1 : Outport
  wires:
  Fcn/1 -> Out1/1
  Sigmoidal MF/1 -> Fcn/1
  "Leaky-Integrator Striatum D1 "/1 -> Sigmoidal MF/1
  In1/1 -> "Leaky-Integrator Striatum D1 "/1

== system BGOnly2/BASAL GANGLIA WITH 5 CHANNELS COMPETITION/Striatum D2/Striatum D2 /StrSat2 ==
  In1 : Inport
  Fcn : Fcn  Expr=u^(1/nu_str)
  "Leaky-Integrator Striatum D1 " : ZeroPole  Zeros=[]  Poles=[-1/teta]  Gain=[1.5/teta]
  Sigmoidal MF : fuzblock/Membership  Functions/Sigmoidal MF  a=alpha_str  c=beta_str_ch(3)
      settings: SourceProductName=Fuzzy Logic Toolbox  SourceProductBaseCode=FL
  Out1 : Outport
  wires:
  Fcn/1 -> Out1/1
  Sigmoidal MF/1 -> Fcn/1
  "Leaky-Integrator Striatum D1 "/1 -> Sigmoidal MF/1
  In1/1 -> "Leaky-Integrator Striatum D1 "/1

== system BGOnly2/BASAL GANGLIA WITH 5 CHANNELS COMPETITION/Striatum D2/Striatum D2 /StrSat3 ==
  In1 : Inport
  Fcn : Fcn  Expr=u^(1/nu_str)
  "Leaky-Integrator Striatum D1 " : ZeroPole  Zeros=[]  Poles=[-1/teta]  Gain=[1.5/teta]
  Sigmoidal MF : fuzblock/Membership  Functions/Sigmoidal MF  a=alpha_str  c=beta_str_ch(4)
      settings: SourceProductName=Fuzzy Logic Toolbox  SourceProductBaseCode=FL
  Out1 : Outport
  wires:
  Fcn/1 -> Out1/1
  Sigmoidal MF/1 -> Fcn/1
  "Leaky-Integrator Striatum D1 "/1 -> Sigmoidal MF/1
  In1/1 -> "Leaky-Integrator Striatum D1 "/1

== system BGOnly2/BASAL GANGLIA WITH 5 CHANNELS COMPETITION/Striatum D2/Striatum D2 /StrSat4 ==
  In1 : Inport
  Fcn : Fcn  Expr=u^(1/nu_str)
  "Leaky-Integrator Striatum D1 " : ZeroPole  Zeros=[]  Poles=[-1/teta]  Gain=[1.5/teta]
  Sigmoidal MF : fuzblock/Membership  Functions/Sigmoidal MF  a=alpha_str  c=beta_str_ch(5)
      settings: SourceProductName=Fuzzy Logic Toolbox  SourceProductBaseCode=FL
  Out1 : Outport
  wires:
  Fcn/1 -> Out1/1
  Sigmoidal MF/1 -> Fcn/1
  "Leaky-Integrator Striatum D1 "/1 -> Sigmoidal MF/1
  In1/1 -> "Leaky-Integrator Striatum D1 "/1

== system BGOnly2/BASAL GANGLIA WITH 5 CHANNELS COMPETITION/SubThalamic Nuclei/SubThalamic Nucleus (STN) /StnSat ==
  In1 : Inport
  Fcn : Fcn  Expr=u^(1/nu_stn)
  "Leaky-Integrator Striatum D1 " : ZeroPole  Zeros=[]  Poles=[-1/teta]  Gain=[1.5/teta]
  Sigmoidal MF : fuzblock/Membership  Functions/Sigmoidal MF  a=alpha_stn  c=beta_stn
      settings: SourceProductName=Fuzzy Logic Toolbox  SourceProductBaseCode=FL
  Out1 : Outport
  wires:
  Fcn/1 -> Out1/1
  Sigmoidal MF/1 -> Fcn/1
  "Leaky-Integrator Striatum D1 "/1 -> Sigmoidal MF/1
  In1/1 -> "Leaky-Integrator Striatum D1 "/1

== system BGOnly2/BASAL GANGLIA WITH 5 CHANNELS COMPETITION/SubThalamic Nuclei/SubThalamic Nucleus (STN) /StnSat1 ==
  In1 : Inport
  Fcn : Fcn  Expr=u^(1/nu_stn)
  "Leaky-Integrator Striatum D1 " : ZeroPole  Zeros=[]  Poles=[-1/teta]  Gain=[1.5/teta]
  Sigmoidal MF : fuzblock/Membership  Functions/Sigmoidal MF  a=alpha_stn  c=beta_stn
      settings: SourceProductName=Fuzzy Logic Toolbox  SourceProductBaseCode=FL
  Out1 : Outport
  wires:
  Fcn/1 -> Out1/1
  Sigmoidal MF/1 -> Fcn/1
  "Leaky-Integrator Striatum D1 "/1 -> Sigmoidal MF/1
  In1/1 -> "Leaky-Integrator Striatum D1 "/1

== system BGOnly2/BASAL GANGLIA WITH 5 CHANNELS COMPETITION/SubThalamic Nuclei/SubThalamic Nucleus (STN) /StnSat2 ==
  In1 : Inport
  Fcn : Fcn  Expr=u^(1/nu_stn)
  "Leaky-Integrator Striatum D1 " : ZeroPole  Zeros=[]  Poles=[-1/teta]  Gain=[1.5/teta]
  Sigmoidal MF : fuzblock/Membership  Functions/Sigmoidal MF  a=alpha_stn  c=beta_stn
      settings: SourceProductName=Fuzzy Logic Toolbox  SourceProductBaseCode=FL
  Out1 : Outport
  wires:
  Fcn/1 -> Out1/1
  Sigmoidal MF/1 -> Fcn/1
  "Leaky-Integrator Striatum D1 "/1 -> Sigmoidal MF/1
  In1/1 -> "Leaky-Integrator Striatum D1 "/1

== system BGOnly2/BASAL GANGLIA WITH 5 CHANNELS COMPETITION/SubThalamic Nuclei/SubThalamic Nucleus (STN) /StnSat3 ==
  In1 : Inport
  Fcn : Fcn  Expr=u^(1/nu_stn)
  "Leaky-Integrator Striatum D1 " : ZeroPole  Zeros=[]  Poles=[-1/teta]  Gain=[1.5/teta]
  Sigmoidal MF : fuzblock/Membership  Functions/Sigmoidal MF  a=alpha_stn  c=beta_stn
      settings: SourceProductName=Fuzzy Logic Toolbox  SourceProductBaseCode=FL
  Out1 : Outport
  wires:
  Fcn/1 -> Out1/1
  Sigmoidal MF/1 -> Fcn/1
  "Leaky-Integrator Striatum D1 "/1 -> Sigmoidal MF/1
  In1/1 -> "Leaky-Integrator Striatum D1 "/1

== system BGOnly2/BASAL GANGLIA WITH 5 CHANNELS COMPETITION/SubThalamic Nuclei/SubThalamic Nucleus (STN) /StnSat4 ==
  In1 : Inport
  Fcn : Fcn  Expr=u^(1/nu_stn)
  "Leaky-Integrator Striatum D1 " : ZeroPole  Zeros=[]  Poles=[-1/teta]  Gain=[1.5/teta]
  Sigmoidal MF : fuzblock/Membership  Functions/Sigmoidal MF  a=alpha_stn  c=beta_stn
      settings: SourceProductName=Fuzzy Logic Toolbox  SourceProductBaseCode=FL
  Out1 : Outport
  wires:
  Fcn/1 -> Out1/1
  Sigmoidal MF/1 -> Fcn/1
  "Leaky-Integrator Striatum D1 "/1 -> Sigmoidal MF/1
  In1/1 -> "Leaky-Integrator Striatum D1 "/1

== matlab function BGOnly2/BASAL GANGLIA WITH 5 CHANNELS COMPETITION/Striatum D2/MATLAB Function ==
  data: ch_in input; ch_out output; w_inhib input
function ch_out = recurrent_inh(ch_in, w_inhib)
    
   ch_out = zeros(1,5);
   for ii = 1:5
        
        kronD = ones(1,5);
        kronD(ii) = 0;
        ch_out(ii) = ch_in(ii) - w_inhib*(sum(ch_in.*kronD'));

   end
end

== matlab function BGOnly2/BASAL GANGLIA WITH 5 CHANNELS COMPETITION/Striatum D1 /MATLAB Function ==
  data: ch_in input; ch_out output; w_inhib input
function ch_out = recurrent_inh(ch_in, w_inhib)
    
   ch_out = zeros(1,5);
   for ii = 1:5
        
        kronD = ones(1,5);
        kronD(ii) = 0;
        ch_out(ii) = ch_in(ii) - w_inhib*(sum(ch_in.*kronD'));

   end
end
